simulink model "reaction_pendulum"  (R2021b)
settings: Solver=FixedStepAuto  StartTime=0.0  StopTime=100  FixedStep=h  RelTol=1e-3  EnableMultiTasking=on
PreLoadFcn:
  | warning('off','MATLAB:dispatcher:InexactMatch');
InitFcn:
  | hwinit
values from neighbouring files (symbols this model uses):
  h = 0.05    [hwinit.m]
  K = dlqr(sys_DT.A,sys_DT.B, Q,R)    [hwinit.m]
  L = place(sys_DT.A', sys_DT.C', p_obsv1)'    [hwinit.m]
  sys_DT = c2d(sys_CT, Ts, 'zoh')    [hwinit.m]
undefined symbols (not defined in the file or in its folder): DiscIntNeverNeededParam, Discrete, Time
libraries: ctrlSharedLib x1, eeLuenbergerObserver x1
settings Model: SimulationMode=external  ExtModeTrigDuration=100000  Creator=user  LastModifiedBy=vgori
settings DataIOCC: SaveFormat=Array  SignalLoggingSaveFormat=ModelDataLogs  SaveOutput=off  SignalLogging=off  DSMLogging=off  SaveTime=off  ReturnWorkspaceOutputs=off
settings OptimizationCC: ExpressionDepthLimit=2147483647  LifeSpan=inf
settings DebuggingCC: UnderspecifiedInitializationDetection=Classic  MergeDetectMultiDrivingBlocksExec=none  SolverPrmCheckMsg=warning  FcnCallInpInsideContextMsg=warning  StateNameClashWarn=warning  SFUnexpectedBacktrackingDiag=warning  SFNoUnconditionalDefaultTransitionDiag=warning  SFExecutionAtInitializationDiag=none  SFMachineParentedDataDiag=warning  ArithmeticOperatorsInVariantConditions=warning
settings HardwareCC: ProdBitPerPointer=32  ProdBitPerSizeT=32  ProdBitPerPtrDiffT=32  ProdLargestAtomicFloat=None  ProdIntDivRoundTo=Undefined  ProdEndianess=Unspecified  ProdWordSize=32  ProdHWDeviceType=32-bit Generic
settings ModelReferenceCC: PropagateSignalLabelsOutOfModel=off
settings SFSimCC: SimUseLocalCustomCode=off  CustomCodeUndefinedFunction=UseInterfaceOnly
settings RTWCC: Description=rpend RTDAC/USB2 (Visual C/C++)  SystemTargetFile=rtcon_rpend_usb2.tlc  TemplateMakefile=rtcon_rpend_vc_usb2_x64.tmf  RTWUseLocalCustomCode=off
settings CodeAppCC: StateflowObjectComments=on
settings STFCustomTargetCC: ModelReferenceCompliant=off  CombineOutputUpdateFcns=on  MatFileLogging=on  GRTInterface=off  SystemTargetFile=rtcon_rpend_usb2.tlc
settings GRTTargetCC: TargetLangStandard=C89/C90 (ANSI)  ModelReferenceCompliant=off  ParMdlRefBuildCompliant=off  CompOptLevelCompliant=off  ConcurrentExecutionCompliant=off  CPPClassGenCompliant=off  UseToolchainInfoCompliant=off  ExtMode=on  ExtModeMexFile=rtcon_ext_comm
settings ConfigComp: CovMetricSettings=dw  CovSaveCumulativeToWorkspaceVar=on  CovSaveSingleToWorkspaceVar=on  CovExternalEMLEnable=off  CovSFcnEnable=off

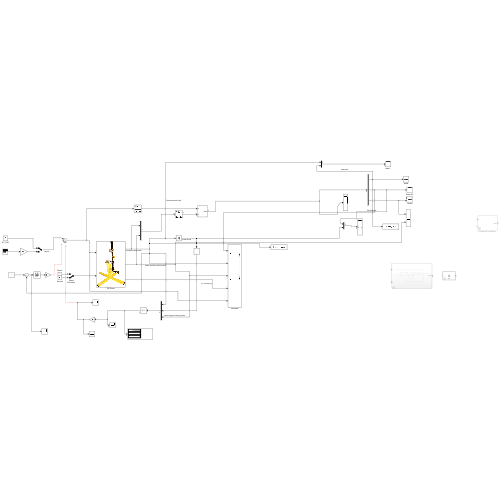
[thumbnail: Simulink's stored preview of the top-level diagram]
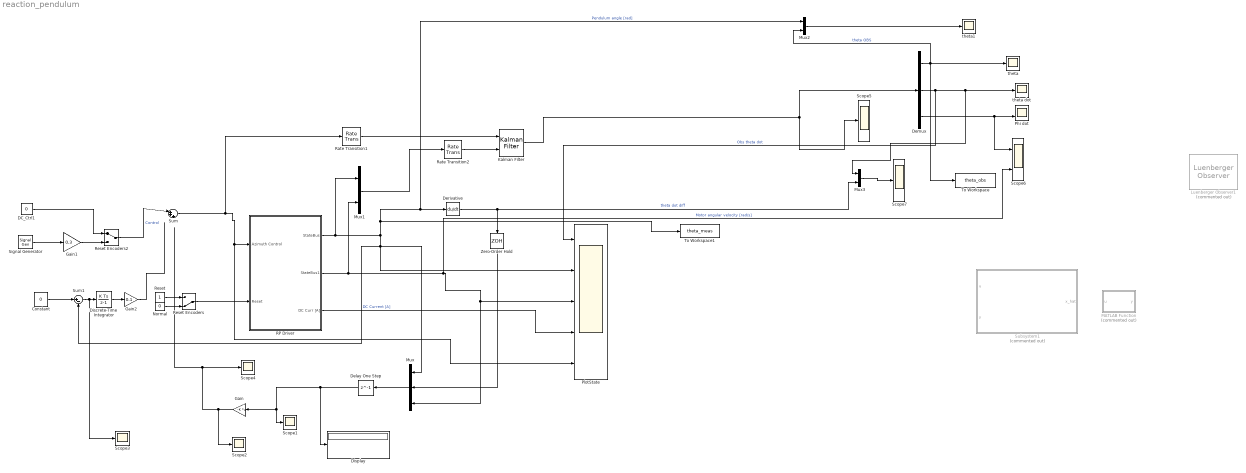
== system reaction_pendulum ==
  Constant : Constant  Value=0
  DC_Ctrl1 : Constant  Value=0
  Delay One Step : Delay  DelayLength=1  SampleTime=h
  Demux : Demux  Outputs=3
  Derivative : Derivative
  Discrete-Time Integrator : DiscreteIntegrator  SampleTime=h  ICPrevOutput=DiscIntNeverNeededParam  ICPrevScaledInput=DiscIntNeverNeededParam
  Display : Display
  Gain : Gain  Gain=-K  Multiplication=Matrix(K*u)
  Gain1 : Gain  Gain=0.3
  Gain2 : Gain  Gain=0.1
  Kalman Filter : ctrlSharedLib/Kalman Filter  TimeDomain=Discrete-Time  UseCurrentEstimator=on  ModelSource=Individual A, B, C, D matrices  ModelSourceVariable=ss(0.95,1,1,0,1)  A=sys_DT.A  B=sys_DT.B  C=sys_DT.C  D=sys_DT.D  NumberOfStates=1  NumberOfInputs=1  NumberOfOutputs=1  InitialEstimateSource=Dialog  X0=[0;0;0]  P0=10  UseK=off  UseGH=off  NumberOfProcessNoiseInputs=1  G=1  TimeInvariantG=on  H=0  TimeInvariantH=on  Q=[1 0 0;0 1000000 0; 0 0 1]  TimeInvariantQ=on  R=1e-5*eye(2)  TimeInvariantR=on  N=0  TimeInvariantN=on  AddInputPort=on  AddEnablePort=off  OutputEstimatedY=off  OutputP=off  Ts=h
  Luenberger Observer1 : eeLuenbergerObserver/Luenberger Observer  Commented=on  StateSpaceType=Discrete-time  Ad=sys_DT.A  Bd=sys_DT.B  Cd=sys_DT.C  Dd=sys_DT.D  A=1  B=1  C=1  D=1  ObserverDesign=Observer gain  Ld=L  DesiredEigenvalues=0  x0=[0 0 0]  Tsd=0.1  Ts=h
      settings: SourceProductBaseCode=PS
  MATLAB Function : MATLAB Function  Commented=on  TreatAsAtomicUnit=on
  Mux : Mux  Inputs=3
  Mux1 : Mux  Inputs=2
  Mux2 : Mux  Inputs=2
  Mux3 : Mux  Inputs=2
  Normal : Constant  Value=0
  Phi dot : Scope  NumInputPorts=2
  PlotState : Scope  NumInputPorts=5
  RP Driver : Subsystem
      mask Display: image(imread('rwp.JPG'))
  Rate Transition1 : RateTransition
  Rate Transition2 : RateTransition
  Reset : Constant
  Reset Encoders : ManualSwitch  CurrentSetting=0
  Reset Encoders2 : ManualSwitch
  Scope{1..5,7} (6 alike) : Scope
  Scope6 : Scope  NumInputPorts=2
  Signal Generator : SignalGenerator  Frequency=1/2
  Subsystem1 : Subsystem  Commented=on
  Sum : Sum  Inputs=|+++
  Sum1 : Sum  Inputs=|+-
  To Workspace : ToWorkspace  VariableName=theta_obs  SaveFormat=Timeseries  SampleTime=-1
  To Workspace1 : ToWorkspace  VariableName=theta_meas  SaveFormat=Timeseries  SampleTime=-1
  Zero-Order Hold : ZeroOrderHold  SampleTime=-1
  theta : Scope
  theta dot : Scope
  theta1 : Scope
  wires:
  Normal/1 -> Reset Encoders/2
  Reset/1 -> Reset Encoders/1
  Reset Encoders/1 -> RP Driver/2(Reset)
  RP Driver/3(DC Curr [A]) -> PlotState/4  "DC Current [A]"
  Reset Encoders2/1 -> Sum/1  "Control"
  DC_Ctrl1/1 -> Reset Encoders2/1
  Signal Generator/1 -> Gain1/1
  RP Driver/2(StateBus1) -> Mux1/2, Scope6/2, Mux/3, PlotState/3  "Motor angular velocity [rad/s]"
  Gain1/1 -> Reset Encoders2/2
  Mux/1 -> Delay One Step/1
  Gain/1 -> Scope4/1, Scope2/1
  Sum1/1 -> Scope3/1, Discrete-Time Integrator/1
  Discrete-Time Integrator/1 -> Gain2/1
  Gain2/1 -> ?
  Constant/1 -> Sum1/1
  Delay One Step/1 -> Display/1, Gain/1, Scope1/1
  RP Driver/1(StateBus) -> Mux1/1, PlotState/2, Mux/1, Sum1/2, Mux2/1, Derivative/1, To Workspace1/1  "Pendulum angle [rad]"
  Kalman Filter/1 -> Scope5/1, Demux/1
  Demux/3 -> Scope6/1, Phi dot/2
  Demux/2 -> Mux3/1, theta dot/1, PlotState/1  "Obs theta dot"
  Demux/1 -> Mux2/2, theta/1, To Workspace/1  "theta OBS"
  Sum/1 -> Rate Transition1/1, PlotState/5, RP Driver/1(Azimuth Control)
  Mux2/1 -> theta1/1
  Mux3/1 -> Scope7/1
  Derivative/1 -> Zero-Order Hold/1, Mux3/2  "theta dot diff"
  Zero-Order Hold/1 -> Mux/2
  Rate Transition2/1 -> Kalman Filter/2
  Mux1/1 -> Rate Transition2/1
  Rate Transition1/1 -> Kalman Filter/1

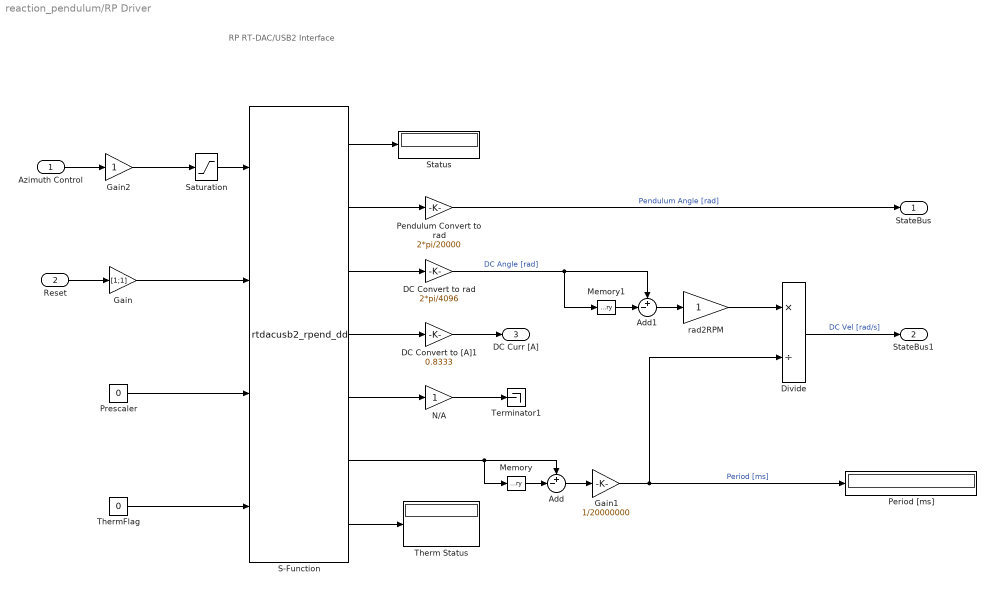
== system reaction_pendulum/RP Driver ==
  note: RP RT-DAC/USB2
      | Interface
  Azimuth Control : Inport
  Reset : Inport  Port=2
  Add : Sum  Inputs=+-|
  Add1 : Sum  Inputs=+-|
  DC Convert to [A]1 : Gain  Gain=0.8333  SaturateOnIntegerOverflow=on  OutDataTypeStr=Inherit: Same as input  ParamDataTypeStr=Inherit: Same as input
  DC Convert to rad : Gain  Gain=2*pi/4096  SaturateOnIntegerOverflow=on  OutDataTypeStr=Inherit: Same as input  ParamDataTypeStr=Inherit: Same as input
  Divide : Product  Inputs=*/
  Gain : Gain  Gain=[1;1]
  Gain1 : Gain  Gain=1/20000000
  Gain2 : Gain
  Memory : Memory
  Memory1 : Memory
  N/A : Gain  SaturateOnIntegerOverflow=on  OutDataTypeStr=Inherit: Same as input  ParamDataTypeStr=Inherit: Same as input
  Pendulum Convert to rad : Gain  Gain=2*pi/20000  SaturateOnIntegerOverflow=on  OutDataTypeStr=Inherit: Same as input  ParamDataTypeStr=Inherit: Same as input
  Period [ms] : Display
  Prescaler : Constant  Value=0
  S-Function : S-Function  FunctionName=rtdacusb2_rpend_dd  Parameters=1, h  SFunctionDeploymentMode=off  EnableBusSupport=off
  Saturation : Saturate  UpperLimit=1  LowerLimit=-1
  Status : Display
  Terminator1 : Terminator
  Therm Status : Display
  ThermFlag : Constant  Value=0
  rad2RPM : Gain  SaturateOnIntegerOverflow=on  OutDataTypeStr=Inherit: Same as input  ParamDataTypeStr=Inherit: Same as input
  StateBus : Outport  VectorParamsAs1DForOutWhenUnconnected=off
  StateBus1 : Outport  Port=2  VectorParamsAs1DForOutWhenUnconnected=off
  DC Curr [A] : Outport  Port=3  VectorParamsAs1DForOutWhenUnconnected=off
  wires:
  S-Function/7 -> Therm Status/1
  S-Function/5 -> N/A/1
  S-Function/4 -> DC Convert to [A]1/1
  ThermFlag/1 -> S-Function/4
  Prescaler/1 -> S-Function/3
  Gain/1 -> S-Function/2
  DC Convert to [A]1/1 -> DC Curr [A]/1
  Divide/1 -> StateBus1/1  "DC Vel [rad/s]"
  rad2RPM/1 -> Divide/1
  Add1/1 -> rad2RPM/1
  Memory1/1 -> Add1/2
  N/A/1 -> Terminator1/1
  S-Function/6 -> Add/1, Memory/1
  Gain2/1 -> Saturation/1
  Gain1/1 -> Period [ms]/1, Divide/2  "Period [ms]"
  Add/1 -> Gain1/1
  Memory/1 -> Add/2
  DC Convert to rad/1 -> Add1/1, Memory1/1  "DC Angle [rad]"
  S-Function/3 -> DC Convert to rad/1
  Pendulum Convert to rad/1 -> StateBus/1  "Pendulum Angle [rad]"
  S-Function/2 -> Pendulum Convert to rad/1
  S-Function/1 -> Status/1
  Saturation/1 -> S-Function/1
  Reset/1 -> Gain/1
  Azimuth Control/1 -> Gain2/1

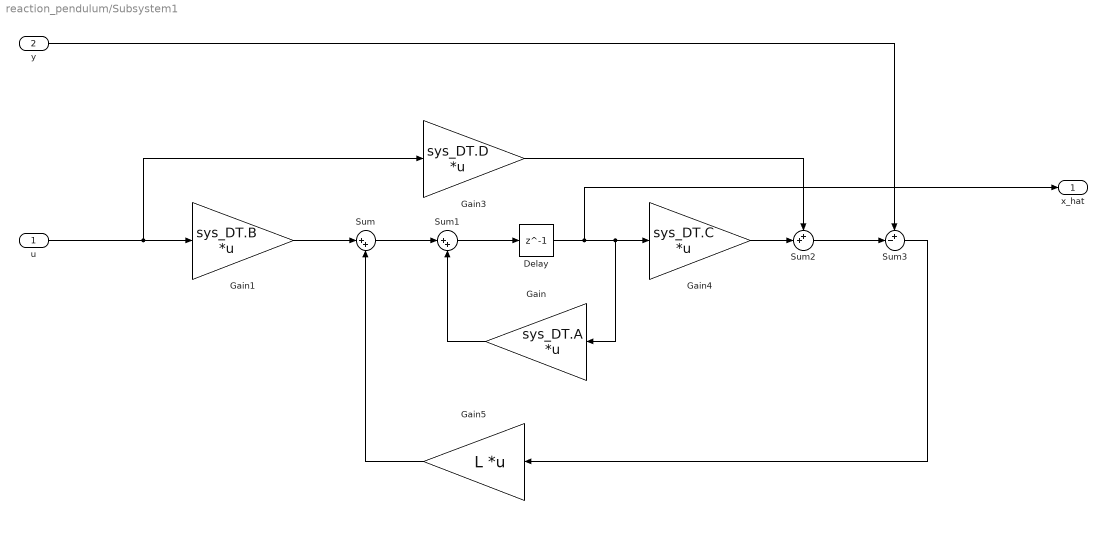
== system reaction_pendulum/Subsystem1 ==
  u : Inport
  y : Inport  Port=2
  Delay : Delay  DelayLength=1  SampleTime=h
  Gain : Gain  Gain=sys_DT.A  Multiplication=Matrix(K*u)
  Gain1 : Gain  Gain=sys_DT.B  Multiplication=Matrix(K*u)
  Gain3 : Gain  Gain=sys_DT.D  Multiplication=Matrix(K*u)
  Gain4 : Gain  Gain=sys_DT.C  Multiplication=Matrix(K*u)
  Gain5 : Gain  Gain=L  Multiplication=Matrix(K*u)
  Sum : Sum  Inputs=|++
  Sum1 : Sum  Inputs=|++
  Sum2 : Sum  Inputs=++|
  Sum3 : Sum  Inputs=+-|
  x_hat : Outport
  wires:
  y/1 -> Sum3/1
  Gain3/1 -> Sum2/1
  Sum2/1 -> Sum3/2
  Gain5/1 -> Sum/2
  Sum3/1 -> Gain5/1
  Gain/1 -> Sum1/2
  Gain4/1 -> Sum2/2
  Sum1/1 -> Delay/1
  Delay/1 -> Gain4/1, Gain/1, x_hat/1
  Sum/1 -> Sum1/1
  Gain1/1 -> Sum/1
  u/1 -> Gain1/1, Gain3/1

== matlab function reaction_pendulum/MATLAB Function ==
  data: u input; y output
function y = fcn(u)
a21 = -9.9834;
a22 = -9.9834;
a24 = 0.0108;
a41 = 11.4724;
a42 = -0.0378;
a44 = -0.9255;
b2  = -3.0625;
b4  = 348.4161;
Ts = 0.05;

A = [0 1 0; 
     -a21 a22 a24; 
     -a41 a42 a44];
B = [0; b2; b4];
C = [1 0 0;
    0 0 1];
D = [0;0];

% Discretize system using 'zoh'
sys_CT = ss(A,B,C,D);
sys_DT = c2d(sys_CT, Ts, 'zoh');

Ts = 0.05;
G_disc = ss(sys_DT.A, sys_DT.B, sys_DT.C, sys_DT.D, Ts);
G_cont = ss(A,B,C,D);
x_hat = (sys_DT.A - L * sys_DT.C) * x_hat + sys_DT.B*u + L*y
y = u;
